simulink library "FAM_quasi_static_outflow"  (R2024a)
settings: Solver=VariableStepAuto  StartTime=0.0  StopTime=10.0  RelTol=1e-3
undefined symbols (not defined in the file): G, power_avg_start_time
libraries: simulink x1
settings Model: Creator=Carson  LastModifiedBy=cmmcguir
settings RTWCC: GPUComputeCapability=3.5

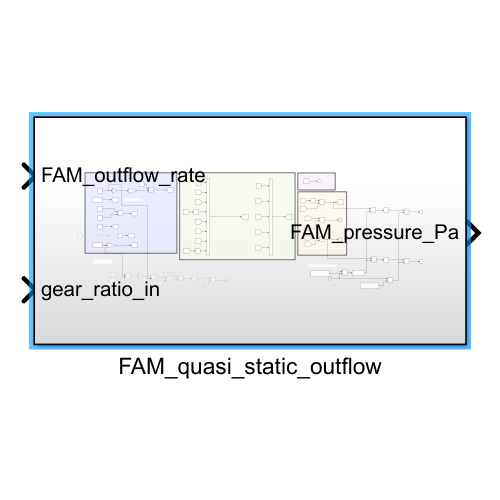
[thumbnail: Simulink's stored preview of the top-level diagram]
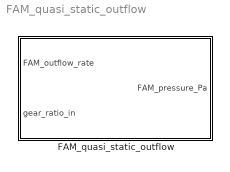
== system FAM_quasi_static_outflow ==
  FAM_quasi_static_outflow : Subsystem

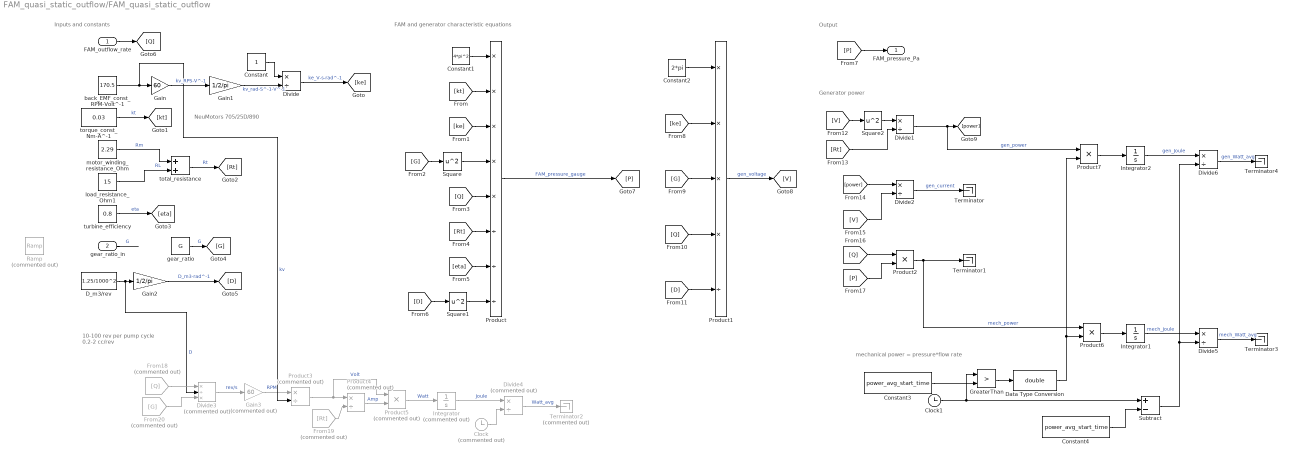
== system FAM_quasi_static_outflow/FAM_quasi_static_outflow ==
  note: NeuMotors 705/25D/890
  note: mechanical power = pressure*flow rate
  note: 10-100 rev per pump cycle
      | 0.2-2 cc/rev
  note: Generator power
  note: Output
  note: FAM and generator characteristic equations
  note: Inputs and constants
  FAM_outflow_rate : Inport
  gear_ratio_in : Inport  Port=2
  Clock : Clock  Commented=on
  Clock1 : Clock
  Constant : Constant
  Constant1 : Constant  Value=4*pi^2
  Constant2 : Constant  Value=2*pi
  Constant3 : Constant  Value=power_avg_start_time
  Constant4 : Constant  Value=power_avg_start_time
  D_m3/rev : Constant  Value=1.25/1000^2
  Data Type Conversion : DataTypeConversion  OutDataTypeStr=double  SaturateOnIntegerOverflow=off  RndMeth=Floor
  Divide{,1..2,5..6} (5 alike) : Product  Inputs=*/
  Divide3 : Product  Commented=on  Inputs=*/*
  Divide4 : Product  Commented=on  Inputs=*/
  From18 : From  Commented=on  GotoTag=Q
  From19 : From  Commented=on  GotoTag=Rt
  From20 : From  Commented=on  GotoTag=G
  Gain : Gain  Gain=60
  Gain1 : Gain  Gain=1/2/pi
  Gain2 : Gain  Gain=1/2/pi
  Gain3 : Gain  Commented=on  Gain=60
  GreaterThan : RelationalOperator  Operator=>  OutDataTypeStr=boolean  RndMeth=Simplest  InputSameDT=off
  Integrator : Integrator  Commented=on
  Integrator1 : Integrator
  Integrator2 : Integrator
  Product : Product  Inputs=*****///
  Product1 : Product  Inputs=****/
  Product2 : Product
  Product3 : Product  Commented=on  Inputs=*/
  Product4 : Product  Commented=on  Inputs=*/
  Product5 : Product  Commented=on  Inputs=**
  Product6 : Product
  Product7 : Product
  Ramp : simulink/Sources/Ramp  Commented=on  slope=0.1  start=60  InitialOutput=1
  Square : Math  Operator=square
  Square1 : Math  Operator=square
  Square2 : Math  Operator=square
  Subtract : Sum  Inputs=+-
  Terminator{,1,3..4} (4 alike) : Terminator
  Terminator2 : Terminator  Commented=on
  back_EMF_const_RPM-Volt^-1 : Constant  Value=170.5
  gear_ratio : Constant  Value=G
  load_resistance_Ohm1 : Constant  Value=15
  motor_winding_resistance_Ohm : Constant  Value=2.29
  torque_const_Nm-A^-1 : Constant  Value=0.03
  total_resistance : Sum
  turbine_efficiency : Constant  Value=0.8
  FAM_pressure_Pa : Outport
  wires:
  FAM_outflow_rate/1 -> [Q]
  torque_const_Nm-A^-1/1 -> [kt]  "kt"
  turbine_efficiency/1 -> [eta]  "eta"
  gear_ratio_in/1 -> ?  "G"
  motor_winding_resistance_Ohm/1 -> total_resistance/1  "Rm"
  load_resistance_Ohm1/1 -> total_resistance/2  "RL"
  total_resistance/1 -> [Rt]  "Rt"
  Gain/1 -> Gain1/1  "kv_RPS-V^-1"
  Gain1/1 -> Divide/2  "kv_rad-S^-1-V^-1"
  Constant/1 -> Divide/1
  Divide/1 -> [ke]  "ke_V-s-rad^-1"
  D_m3/rev/1 -> Divide3/2, Gain2/1  "D"
  Gain2/1 -> [D]  "D_m3-rad^-1"
  Constant1/1 -> Product/1
  [kt] -> Product/2
  [ke] -> Product/3
  [G] -> Square/1
  Square/1 -> Product/4
  [Q] -> Product/5
  [Rt] -> Product/6
  [eta] -> Product/7
  [D] -> Square1/1
  Square1/1 -> Product/8
  Product/1 -> [P]  "FAM_pressure_gauge"
  [P] -> FAM_pressure_Pa/1
  Constant2/1 -> Product1/1
  [ke] -> Product1/2
  [G] -> Product1/3
  [Q] -> Product1/4
  [D] -> Product1/5
  Product1/1 -> [V]  "gen_voltage"
  [V] -> Square2/1
  Square2/1 -> Divide1/1
  [Rt] -> Divide1/2
  Divide1/1 -> Product7/1, [power]  "gen_power"
  [power] -> Divide2/1
  [V] -> Divide2/2
  Divide2/1 -> Terminator/1  "gen_current"
  [Q] -> Product2/1
  [P] -> Product2/2
  Product2/1 -> Product6/1, Terminator1/1  "mech_power"
  From18/1 -> Divide3/1
  Divide3/1 -> Gain3/1  "rev/s"
  Gain3/1 -> Product3/1  "RPM"
  back_EMF_const_RPM-Volt^-1/1 -> Product3/2, Gain/1  "kv"
  Product3/1 -> Product5/1, Product4/1  "Volt"
  From19/1 -> Product4/2
  Product4/1 -> Product5/2  "Amp"
  Product5/1 -> Integrator/1  "Watt"
  From20/1 -> Divide3/3
  Integrator/1 -> Divide4/1  "Joule"
  Clock/1 -> Divide4/2
  Divide4/1 -> Terminator2/1  "Watt_avg"
  Divide5/1 -> Terminator3/1  "mech_Watt_avg"
  Integrator1/1 -> Divide5/1  "mech_Joule"
  gear_ratio/1 -> [G]  "G"
  Divide6/1 -> Terminator4/1  "gen_Watt_avg"
  Integrator2/1 -> Divide6/1  "gen_Joule"
  Clock1/1 -> Subtract/1, GreaterThan/1
  GreaterThan/1 -> Data Type Conversion/1
  Constant3/1 -> GreaterThan/2
  Data Type Conversion/1 -> Product6/2, Product7/2
  Product6/1 -> Integrator1/1
  Constant4/1 -> Subtract/2
  Subtract/1 -> Divide6/2, Divide5/2
  Product7/1 -> Integrator2/1
